simulink model "SostituisciScatola"  (R2019a)
settings: Solver=VariableStepAuto  StartTime=0.0  StopTime=10.0  RelTol=1e-3
settings Model: Creator=anton  LastModifiedBy=anton

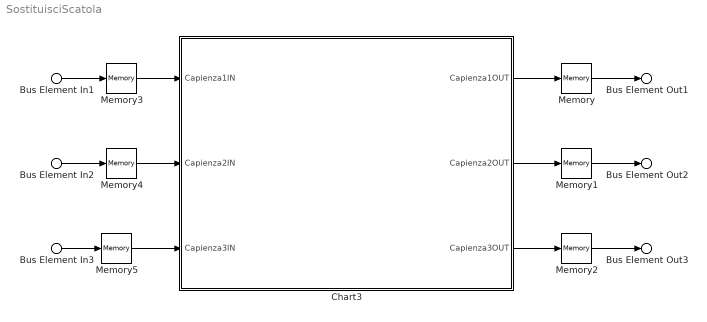
== system SostituisciScatola ==
  Bus Element In1 : Inport  PortName=Capienza1IN
  Bus Element In2 : Inport  Port=2  PortName=Capienza2IN
  Bus Element In3 : Inport  Port=3  PortName=Capienza3IN
  Chart3 : Stateflow chart  BlockKeywords=__PRM__SERIALIZED__DATA__:Stateflow Chart,Stateflow Diagram  TreatAsAtomicUnit=on
  Memory{,1..5} (6 alike) : Memory
  Bus Element Out1 : Outport  PortName=Capienza1OUT
  Bus Element Out2 : Outport  Port=2  PortName=Capienza2OUT
  Bus Element Out3 : Outport  Port=3  PortName=Capienza3OUT
  wires:
  Chart3/1(Capienza1OUT) -> Memory/1
  Memory/1 -> Bus Element Out1/1
  Memory1/1 -> Bus Element Out2/1
  Chart3/2(Capienza2OUT) -> Memory1/1
  Chart3/3(Capienza3OUT) -> Memory2/1
  Memory2/1 -> Bus Element Out3/1
  Memory5/1 -> Chart3/3(Capienza3IN)
  Bus Element In3/1 -> Memory5/1
  Bus Element In2/1 -> Memory4/1
  Memory4/1 -> Chart3/2(Capienza2IN)
  Bus Element In1/1 -> Memory3/1
  Memory3/1 -> Chart3/1(Capienza1IN)

== stateflow chart SostituisciScatola/Chart3 ==
  state Idle
    Capienza1OUT=0;
    Capienza2OUT=0;
    Capienza3OUT=0;
  state Scatola1Expired
    Capienza1OUT=1;
  state Scatola2Expired
    Capienza2OUT=1;
  state Scatola3Expired
    Capienza3OUT=1;
  (default) -> Idle
  Idle -> Scatola1Expired [order 1] : [Capienza1IN<=0]
  Idle -> Scatola3Expired [order 3] : [Capienza3IN>=6]
  Scatola3Expired -> Idle
  Scatola1Expired -> Idle
  Scatola2Expired -> Idle
  Idle -> Scatola2Expired [order 2] : [Capienza2IN<=0]
  data: Capienza1IN input; Capienza2IN input; Capienza3IN input; Capienza1OUT output; Capienza2OUT output; Capienza3OUT output
